simulink model "UNICO"  (R2023b)
settings: Solver=FixedStepDiscrete  StartTime=0.0  StopTime=inf  FixedStep=Control.DT  RelTol=1e-3
values from neighbouring files (symbols this model uses):
  Control =     [Parameters_UNICO.mat]
libraries: simulink x2
(part 3 of 3)

== matlab function UNICO/Wind Speed Estimators/Extended Kalman Filter/GenSpeed_input ==
  data: GenSpMin input; we_inp_speed output; Gearbox_ratio input; RotorSpeed input
function we_inp_speed = fcn(GenSpMin,Gearbox_ratio,RotorSpeed)
% Function to ensure the rotor speed does not fall below a minimum threshold

if RotorSpeed < 0.25*GenSpMin/Gearbox_ratio         % Check if the rotor speed is below 25% of the minimum generator speed, adjusted by the gearbox ratio
    
    we_inp_speed = 0.25*GenSpMin/Gearbox_ratio;     % Set the input speed to the minimum allowable value

else                                                % Otherwise, use the actual rotor speed

    we_inp_speed = RotorSpeed;

end

end

== matlab function UNICO/Pitch Rate Limiter/Rate limiter ==
  data: u_b input; u input; s output; Pitch_Rate input; dt input
function s = fcn(u_b,u,Pitch_Rate, dt)

rate_lim_pos = Pitch_Rate; % rate limit for pitch is simmetric
rate_lim_neg = -Pitch_Rate;

% calculate pitch rate
rate = (u-u_b)/dt;

if rate > rate_lim_pos % if the pitch rate is larger than the maximum allowed, set the pitch using the maximum rate

    s = u_b+rate_lim_pos*dt;

elseif rate < rate_lim_neg % if the pitch rate is smaller than the minimum allowed, set the pitch using the minimum rate

    s = u_b+rate_lim_neg*dt;

else

    s = u;  % if the maximum pitch rate is not violated

end

== matlab function UNICO/Wind Speed Estimators/Extended Kalman Filter/Torque_input ==
  data: GenTorque input; input_torque output; rated_torque input
function input_torque = fcn(GenTorque,rated_torque)
% Function to limit the generator torque to a minimum threshold

if GenTorque < 0.001*rated_torque               % If the generator torque is below 0.001 times the rated torque
    
    input_torque = 0.001*rated_torque;          % Set the input torque to the minimum allowable value

else                                            % Otherwise, use the actual generator torque

    input_torque = GenTorque;

end

end

== matlab function UNICO/Wind Speed Estimators/MATLAB Function ==
  data: WSE_Mode input; TBE_WSpeed input; Raw_WSpeed input; WSpeed output; EKF_WSpeed input
function WSpeed = fcn(WSE_Mode, TBE_WSpeed, Raw_WSpeed, EKF_WSpeed)
if WSE_Mode == 1
    WSpeed = TBE_WSpeed;
elseif WSE_Mode == 2
    WSpeed = EKF_WSpeed;
else
    WSpeed = Raw_WSpeed;
end

== matlab function UNICO/Set Point Smoother/GenSpeed_Ref_Torque_Controller ==
  data: Gen_Ref_torq input; delta_omega input; y output
function y = fcn(Gen_Ref_torq, delta_omega)
% Defining the new generator speed reference for the torque controller

if delta_omega >= 0                     % In Region 2.5 and 3 modify the reference generator speed to avoid conflict with pitch controller

    y = Gen_Ref_torq - delta_omega;     % Following Abbas's rules

else                                    % In Region 2 do no modify the reference generator speed

    y = Gen_Ref_torq;                   

end

end

== matlab function UNICO/Wind Speed Estimators/Extended Kalman Filter/MATLAB Function2 ==
  data: params input; Rot_In output; Radius output; Blade_Height output; Air_Density output; Gearbox_Ratio output; Rated_Torque output; Minimum_Rot_Speed output; Rotor_Area output
function [Rot_In, Radius, Blade_Height, Air_Density, Gearbox_Ratio, Rated_Torque, Minimum_Rot_Speed, Rotor_Area] = fcn(params)
% extracting the generator speed reference   
Radius = params(1); 
Air_Density = params(22);
Blade_Height = params(24);
Rot_In = params(25);
Gearbox_Ratio = params(27);
Rotor_Area = params(28);
Rated_Torque = params(3);
Minimum_Rot_Speed = params(9);
end

== matlab function UNICO/Extract Signals & Filtering/Filtering Block  ==
  data: windNF input; wnd output; wind input; GenSpeedNF input; GenSpeed input; Pitch input; PitchNF input; Tq input; TqNF input; Pwr input; PwrNF input; time input; omega output; ptch output; torque output; Power output; LPF_Starting_Time input
function [wnd,omega,ptch,torque,Power] = fcn(windNF, wind,GenSpeedNF, GenSpeed, Pitch, PitchNF, Tq, TqNF, Pwr, PwrNF, time, LPF_Starting_Time)

% At the beginning of the simulation do not apply filtering to avoid divergence

if time > LPF_Starting_Time

    wnd=wind;        % Wind speed filtered

    omega=GenSpeed;  % Generator speed filtered

    ptch=Pitch;      % Blade picth angle filtered

    torque=Tq;       % Generator torque filtered

    Power=Pwr;       % Generator power filtered

else

    wnd=windNF;         % Wind speed unfiltered

    omega=GenSpeedNF;   % Generator speed unfiltered

    ptch=PitchNF;       % Blade picth angle unfiltered

    torque=TqNF;        % Generator torque unfiltered

    Power=PwrNF;        % Generator power unfiltered

end

== matlab function UNICO/Wind Speed Estimators/Torque Balance Estimator/MATLAB Function2 ==
  data: params input; Rot_In output; Radius output; Blade_Height output; Air_Density output; Gearbox_Ratio output; Rotor_Area output
function [Rot_In, Radius, Blade_Height, Air_Density, Gearbox_Ratio, Rotor_Area]    = fcn(params)
% extracting the generator speed reference 
Radius = params(1); 
Rot_In = params(25);
Blade_Height = params(24);
Air_Density = params(22);
Gearbox_Ratio = params(27);
Rotor_Area = params(28);

end

== matlab function UNICO/Reference Speed Determination/MATLAB Function ==
  data: w0 input; freq input; Ts input; u input; y output
function y = discreteVaryingLowpass(w0, freq, Ts, u)
% DISCRETEVARYINGLOWPASS Implements a 1st-order variable Butterworth filter.
%
% INPUTS:
%   u    : Current input signal
%   freq : Cutoff frequency in rad/s (can vary at each step)
%   Ts   : Sample time in seconds
%   w0   : Pre-warping frequency (rad/s). Set to 0 for standard Tustin.
%
% OUTPUT:
%   y    : Filtered output signal

    % Persistent variables to maintain state between time steps
    persistent u_prev y_prev
    
    % Initialization on the first run
    if isempty(u_prev)
        u_prev = u;
        y_prev = u;
    end

    % --- 1. Pre-warping Gain (K) ---
    % Standard Bilinear (Tustin) transform uses K = 2/Ts.
    % If a pre-warping frequency w0 is provided, K is adjusted.
    if w0 <= 0
        K = 2 / Ts;
    else
        K = w0 / tan(w0 * Ts / 2);
    end

    % --- 2. Variable Coefficient Calculation ---
    % Continuous Transfer Function: H(s) = freq / (s + freq)
    % Substitution: s = K * (z-1) / (z+1)
    
    denominator = (K + freq);
    b0 = freq / denominator;
    b1 = b0;                     % For 1st order Tustin, b0 always equals b1
    a1 = (freq - K) / denominator;

    % --- 3. Difference Equation ---
    % Standard Direct Form I implementation:
    % y[n] = b0*u[n] + b1*u[n-1] - a1*y[n-1]
    y = b0*u + b1*u_prev - a1*y_prev;

    % --- 4. State Update ---
    u_prev = u;
    y_prev = y;
end

== matlab function UNICO/Wind Speed Estimators/Torque Balance Estimator/Torque Balance Estimator LPF ==
  data: w0 input; freq input; Ts input; u input; y output
function y = discreteVaryingLowpass(w0, freq, Ts, u)
% DISCRETEVARYINGLOWPASS Implements a 1st-order variable Butterworth filter.
%
% INPUTS:
%   u    : Current input signal
%   freq : Cutoff frequency in rad/s (can vary at each step)
%   Ts   : Sample time in seconds
%   w0   : Pre-warping frequency (rad/s). Set to 0 for standard Tustin.
%
% OUTPUT:
%   y    : Filtered output signal

    % Persistent variables to maintain state between time steps
    persistent u_prev y_prev
    
    % Initialization on the first run
    if isempty(u_prev)
        u_prev = 0;
        y_prev = 0;
    end

    % --- 1. Pre-warping Gain (K) ---
    % Standard Bilinear (Tustin) transform uses K = 2/Ts.
    % If a pre-warping frequency w0 is provided, K is adjusted.
    if w0 <= 0
        K = 2 / Ts;
    else
        K = w0 / tan(w0 * Ts / 2);
    end

    % --- 2. Variable Coefficient Calculation ---
    % Continuous Transfer Function: H(s) = freq / (s + freq)
    % Substitution: s = K * (z-1) / (z+1)
    
    denominator = (K + freq);
    b0 = freq / denominator;
    b1 = b0;                     % For 1st order Tustin, b0 always equals b1
    a1 = (freq - K) / denominator;

    % --- 3. Difference Equation ---
    % Standard Direct Form I implementation:
    % y[n] = b0*u[n] + b1*u[n-1] - a1*y[n-1]
    y = b0*u + b1*u_prev - a1*y_prev;

    % --- 4. State Update ---
    u_prev = u;
    y_prev = y;
end

== matlab function UNICO/Wind Speed Estimators/Extended Kalman Filter/Extended Kalman Filter LPF ==
  data: w0 input; freq input; Ts input; u input; y output
function y = discreteVaryingLowpass(w0, freq, Ts, u)
% DISCRETEVARYINGLOWPASS Implements a 1st-order variable Butterworth filter.
%
% INPUTS:
%   u    : Current input signal
%   freq : Cutoff frequency in rad/s (can vary at each step)
%   Ts   : Sample time in seconds
%   w0   : Pre-warping frequency (rad/s). Set to 0 for standard Tustin.
%
% OUTPUT:
%   y    : Filtered output signal

    % Persistent variables to maintain state between time steps
    persistent u_prev y_prev
    
    % Initialization on the first run
    if isempty(u_prev)
        u_prev = 0;
        y_prev = 0;
    end

    % --- 1. Pre-warping Gain (K) ---
    % Standard Bilinear (Tustin) transform uses K = 2/Ts.
    % If a pre-warping frequency w0 is provided, K is adjusted.
    if w0 <= 0
        K = 2 / Ts;
    else
        K = w0 / tan(w0 * Ts / 2);
    end

    % --- 2. Variable Coefficient Calculation ---
    % Continuous Transfer Function: H(s) = freq / (s + freq)
    % Substitution: s = K * (z-1) / (z+1)
    
    denominator = (K + freq);
    b0 = freq / denominator;
    b1 = b0;                     % For 1st order Tustin, b0 always equals b1
    a1 = (freq - K) / denominator;

    % --- 3. Difference Equation ---
    % Standard Direct Form I implementation:
    % y[n] = b0*u[n] + b1*u[n-1] - a1*y[n-1]
    y = b0*u + b1*u_prev - a1*y_prev;

    % --- 4. State Update ---
    u_prev = u;
    y_prev = y;
end

== matlab function UNICO/Set Point Smoother/MATLAB Function1 ==
  data: w0 input; freq input; Ts input; u input; y output
function y = discreteVaryingLowpass(w0, freq, Ts, u)
% DISCRETEVARYINGLOWPASS Implements a 1st-order variable Butterworth filter.
%
% INPUTS:
%   u    : Current input signal
%   freq : Cutoff frequency in rad/s (can vary at each step)
%   Ts   : Sample time in seconds
%   w0   : Pre-warping frequency (rad/s). Set to 0 for standard Tustin.
%
% OUTPUT:
%   y    : Filtered output signal

    % Persistent variables to maintain state between time steps
    persistent u_prev y_prev
    
    % Initialization on the first run
    if isempty(u_prev)
        u_prev = 0;
        y_prev = 0;
    end

    % --- 1. Pre-warping Gain (K) ---
    % Standard Bilinear (Tustin) transform uses K = 2/Ts.
    % If a pre-warping frequency w0 is provided, K is adjusted.
    if w0 <= 0
        K = 2 / Ts;
    else
        K = w0 / tan(w0 * Ts / 2);
    end

    % --- 2. Variable Coefficient Calculation ---
    % Continuous Transfer Function: H(s) = freq / (s + freq)
    % Substitution: s = K * (z-1) / (z+1)
    
    denominator = (K + freq);
    b0 = freq / denominator;
    b1 = b0;                     % For 1st order Tustin, b0 always equals b1
    a1 = (freq - K) / denominator;

    % --- 3. Difference Equation ---
    % Standard Direct Form I implementation:
    % y[n] = b0*u[n] + b1*u[n-1] - a1*y[n-1]
    y = b0*u + b1*u_prev - a1*y_prev;

    % --- 4. State Update ---
    u_prev = u;
    y_prev = y;
end

== matlab function UNICO/Set Point Smoother/MATLAB Function2 ==
  data: w0 input; freq input; Ts input; u input; y output
function y = discreteVaryingLowpass(w0, freq, Ts, u)
% DISCRETEVARYINGLOWPASS Implements a 1st-order variable Butterworth filter.
%
% INPUTS:
%   u    : Current input signal
%   freq : Cutoff frequency in rad/s (can vary at each step)
%   Ts   : Sample time in seconds
%   w0   : Pre-warping frequency (rad/s). Set to 0 for standard Tustin.
%
% OUTPUT:
%   y    : Filtered output signal

    % Persistent variables to maintain state between time steps
    persistent u_prev y_prev
    
    % Initialization on the first run
    if isempty(u_prev)
        u_prev = 0;
        y_prev = 0;
    end

    % --- 1. Pre-warping Gain (K) ---
    % Standard Bilinear (Tustin) transform uses K = 2/Ts.
    % If a pre-warping frequency w0 is provided, K is adjusted.
    if w0 <= 0
        K = 2 / Ts;
    else
        K = w0 / tan(w0 * Ts / 2);
    end

    % --- 2. Variable Coefficient Calculation ---
    % Continuous Transfer Function: H(s) = freq / (s + freq)
    % Substitution: s = K * (z-1) / (z+1)
    
    denominator = (K + freq);
    b0 = freq / denominator;
    b1 = b0;                     % For 1st order Tustin, b0 always equals b1
    a1 = (freq - K) / denominator;

    % --- 3. Difference Equation ---
    % Standard Direct Form I implementation:
    % y[n] = b0*u[n] + b1*u[n-1] - a1*y[n-1]
    y = b0*u + b1*u_prev - a1*y_prev;

    % --- 4. State Update ---
    u_prev = u;
    y_prev = y;
end

== matlab function UNICO/Reference Speed Determination/MATLAB Function2 ==
  data: SimTime input; params input; RefSpeedFiltered input; RefSpeedUnfiltered input; Genspeed output
function Genspeed = fcn(SimTime, params, RefSpeedFiltered, RefSpeedUnfiltered)
NF_StartingTime = params(11);

if SimTime > NF_StartingTime
Genspeed = RefSpeedFiltered;
else 
Genspeed =  RefSpeedUnfiltered;
end

== matlab function UNICO/MATLAB Function3 ==
  data: w0 input; freq input; Ts input; u input; y output
function y = discreteVaryingLowpass(w0, freq, Ts, u)
% DISCRETEVARYINGLOWPASS Implements a 1st-order variable Butterworth filter.
%
% INPUTS:
%   u    : Current input signal
%   freq : Cutoff frequency in rad/s (can vary at each step)
%   Ts   : Sample time in seconds
%   w0   : Pre-warping frequency (rad/s). Set to 0 for standard Tustin.
%
% OUTPUT:
%   y    : Filtered output signal

    % Persistent variables to maintain state between time steps
    persistent u_prev y_prev
    
    % Initialization on the first run
    if isempty(u_prev)
        u_prev = 0;
        y_prev = 0;
    end

    % --- 1. Pre-warping Gain (K) ---
    % Standard Bilinear (Tustin) transform uses K = 2/Ts.
    % If a pre-warping frequency w0 is provided, K is adjusted.
    if w0 <= 0
        K = 2 / Ts;
    else
        K = w0 / tan(w0 * Ts / 2);
    end

    % --- 2. Variable Coefficient Calculation ---
    % Continuous Transfer Function: H(s) = freq / (s + freq)
    % Substitution: s = K * (z-1) / (z+1)
    
    denominator = (K + freq);
    b0 = freq / denominator;
    b1 = b0;                     % For 1st order Tustin, b0 always equals b1
    a1 = (freq - K) / denominator;

    % --- 3. Difference Equation ---
    % Standard Direct Form I implementation:
    % y[n] = b0*u[n] + b1*u[n-1] - a1*y[n-1]
    y = b0*u + b1*u_prev - a1*y_prev;

    % --- 4. State Update ---
    u_prev = u;
    y_prev = y;
end

== matlab function UNICO/MATLAB Function4 ==
  data: SimTime input; params input; GenTqFiltered input; GenTqUnfiltered input; GenTq output
function GenTq = fcn(SimTime, params, GenTqFiltered, GenTqUnfiltered)
NF_StartingTime = params(11);

if SimTime > NF_StartingTime
GenTq = GenTqFiltered;
else 
GenTq =  GenTqUnfiltered;
end

== matlab function UNICO/Notch Filter/MATLAB Function2 ==
  data: SimTime input; NFparams input; GenSpeedUnfiltered input; GenSpeedFiltered input; Genspeed output
function Genspeed = fcn(SimTime, NFparams, GenSpeedUnfiltered, GenSpeedFiltered)
NF_StartingTime = NFparams;

if SimTime > NF_StartingTime
Genspeed = GenSpeedFiltered;
else 
Genspeed =  GenSpeedUnfiltered;
end

== matlab function UNICO/Notch Filter/MATLAB Function3 ==
  data: u input; Ts input; f0 input; Filt_GenTq output; zeta_z input; zeta_p input
function Filt_GenTq = notch_filter(u, Ts, f0, zeta_z, zeta_p)

persistent x1 x2 y1 y2 last_f0 last_Ts last_zz last_zp ...
           b0 b1 b2 a1 a2

% Initialize on first run
if isempty(x1)
    x1 = u; x2 = u;
    y1 = u; y2 = u;

    last_f0 = -1;
    last_Ts = -1;
    last_zz = -1;
    last_zp = -1;

    b0 = 1; b1 = 0; b2 = 0;
    a1 = 0; a2 = 0;
end

% Recompute coefficients only when parameters change AND Ts > 0
if (f0 ~= last_f0) || (Ts ~= last_Ts) || ...
   (zeta_z ~= last_zz) || (zeta_p ~= last_zp)

    if Ts > 0
        omega0 = 2*pi*f0;
        K  = 2 / Ts;
        K2 = K * K;
        w2 = omega0 * omega0;

        % Bilinear (Tustin) transform — numerator
        bz0 = K2 + 2*zeta_z*omega0*K + w2;
        bz1 = 2*w2 - 2*K2;
        bz2 = K2 - 2*zeta_z*omega0*K + w2;

        % Bilinear (Tustin) transform — denominator
        az0 = K2 + 2*zeta_p*omega0*K + w2;
        az1 = 2*w2 - 2*K2;
        az2 = K2 - 2*zeta_p*omega0*K + w2;

        % Normalize so a[0] = 1
        b0 = bz0 / az0;
        b1 = bz1 / az0;
        b2 = bz2 / az0;
        a1 = az1 / az0;
        a2 = az2 / az0;
    end
    % Always cache the current parameters (even when Ts=0)
    % so the next call (Ts=dt>0) recomputes correctly
    last_f0 = f0;
    last_Ts = Ts;
    last_zz = zeta_z;
    last_zp = zeta_p;
end

% IIR difference equation
Filt_GenTq = b0*u + b1*x1 + b2*x2 - a1*y1 - a2*y2;

% Update delay states
x2 = x1;
x1 = u;
y2 = y1;
y1 = Filt_GenTq;

end

== matlab function UNICO/Pitch Rate Limiter1/Rate limiter ==
  data: u_b input; u input; s output; Pitch_Rate input; dt input
function s = fcn(u_b, u, Pitch_Rate, dt)
% fcn  Pitch rate limiter (symmetric), all quantities in degrees.
%
%   s = fcn(u_b, u, Pitch_Rate, dt)
%
%   u_b         : previous pitch command [deg]
%   u           : desired (unlimited) pitch command [deg]
%   Pitch_Rate  : maximum allowed pitch rate, given in [rad/s] (symmetric, +/-)
%   dt          : sample time [s]
%   s           : rate-limited pitch command [deg]

rate_lim_pos = Pitch_Rate * (180/pi);     % rate limit for pitch is symmetric [deg/s] (converted from rad/s)
rate_lim_neg = -Pitch_Rate * (180/pi);    % [deg/s]

% calculate pitch rate [deg/s]
rate = (u - u_b) / dt;

if rate > rate_lim_pos
    % if the pitch rate is larger than the maximum allowed, set the pitch using the maximum rate
    s = u_b + rate_lim_pos * dt;
elseif rate < rate_lim_neg
    % if the pitch rate is smaller than the minimum allowed, set the pitch using the minimum rate
    s = u_b + rate_lim_neg * dt;
else
    s = u;  % if the maximum pitch rate is not violated
end

end

== matlab function UNICO/PI CONTROLLER/Gain scheduling ==
  data: GenSpeed input; WindSpeed input; kp_ar input; Ki output; ki_ar input; kp_br input; ki_br input; Kp output; Params input
function [Ki,Kp] = fcn(GenSpeed, WindSpeed, kp_ar, ki_ar,kp_br, ki_br, Params)

R       = Params(1);  % Rotor radius           [m]
v_rt    = Params(2);  % Rated power wind speed [m/s]
w_rt    = Params(5);  % Rated generator speed  [rad/s]
r2      = Params(10);  % Region 2 control mode  {0: optimum tsr tracking; 1: kw^2 torque law}
SpdSwitch = Params(13); %generator speed for switch between region 2 and 2 1/2

% if we use TSR tracking in below rated conditions, schedule the PI
% coefficients
if r2 == 0

    if WindSpeed < v_rt && GenSpeed < w_rt

        % if GenSpeed <=SpdSwitch
        if GenSpeed <= SpdSwitch
            Kp = kp_br;
            Ki = ki_br;

        elseif GenSpeed > SpdSwitch && GenSpeed <w_rt
            % else

            Kp = kp_br+(kp_ar-kp_br)/(w_rt-SpdSwitch)*(GenSpeed-SpdSwitch);
            Ki = ki_br+(ki_ar-ki_br)/(w_rt-SpdSwitch)*(GenSpeed-SpdSwitch);

        else

            Kp = kp_ar;
            Ki = ki_ar;
            % end
        end


    else

        Kp = kp_ar;
        Ki = ki_ar;
    end

else
    % if k-w is used only a set of kp and ki is used
    Kp = kp_ar;
    Ki = ki_ar;

end

== matlab function UNICO/MATLAB Function1 ==
  data: Torque_PI_out input; WindSpeed input; dFPitch input; Pitch_Ctrl_Sw input; Pitch_Controller_Out input; Pitch_out output; params input; Torque_out output
function [Pitch_out, Torque_out] = Pitch_Switch(Torque_PI_out, WindSpeed, dFPitch, Pitch_Ctrl_Sw, Pitch_Controller_Out, params)
v_rt  = params(2);                  % Rated power wind speed [m/s]
dRtTq = params(3);                  % Rated Torque [Nm]

if WindSpeed > v_rt
    if Pitch_Ctrl_Sw == 0
        Pitch_out  = dFPitch * (pi / 180);  % deg → rad
        Torque_out = Torque_PI_out;
    else
        Pitch_out  = Pitch_Controller_Out;
        Torque_out = dRtTq;
    end
else
    Pitch_out  = 0;              % sotto v_rt: passo a zero (fine pitch)
    Torque_out = Torque_PI_out;
end

end

== matlab function UNICO/PI CONTROLLER/Initialize integral term ==
  data: checkDelay input; check output; PI_int input; PI_int output; wg input; WindSpeed input; Architecture_Selector input; Darrieus_Selector input; Params input; propTerm input; T_eq output
function [check,PI_int, T_eq] = fcn(checkDelay, PI_int, wg, WindSpeed, Architecture_Selector, Darrieus_Selector, Params, propTerm)
% Load R struct variables
R       = Params(1);  % Rotor radius                       [m]
v_rt    = Params(2);  % Rated power wind speed             [m/s]
Tq_rated = Params(3); % Rated torque                       [Nm]
w_rt    = Params(5);  % Rated generator speed              [rad/s]
w_min   = Params(9);  % Minimum generator speed            [rad/s]
r2      = Params(10); % Region 2 control mode  {0: optimum tsr tracking; 1: kw^2 torque law}
KSwitch = Params(11); % Region 2 K- switch
Rgn2K = Params(12);   % user defined K value
SpdSwitch = Params(13); %generator speed for switch between region 2 and 2 1/2
w_minSwitch = Params(14); % Switch between region 1.5 and 2 [rad/s]
TSR_opt = Params(15);  % Optimum TSR                             [-]
Cpmax   = Params(16); % max cp value                             [-]
rho     = Params(22);  % Air density                             [kg/m^3]
Bld_Height = Params(24); %Blades Height (VAWT ONLY)              [m]
Rot_area= Params(28); % Rotor Area (VAWT Eggbeater Type ONLY) [m^2]

% Calcola K coerentemente con l'architettura (usato in entrambi i rami r2)
if KSwitch == 1
    K = Rgn2K;
else
    if Architecture_Selector == 1
        K = 0.5*rho*pi*R^5*Cpmax/TSR_opt^3;          % HAWT
    else
        if Darrieus_Selector == 1
            K = rho*R^4*Bld_Height*Cpmax/TSR_opt^3;  % VAWT H-type
        else
            K = 0.5*rho*Rot_area*R^3*Cpmax/TSR_opt^3; % VAWT Eggbeater
        end
    end
end

% ===========================================
% PRIMA: Controlla se siamo in Regione 3
% ===========================================
if WindSpeed > v_rt
    check = 3;
    if checkDelay ~= 3
        % Entrando in Regione 3: inizializza per dare Torque = Torque_rated
        PI_int = Tq_rated - propTerm;
    end

% ===========================================
% ALTRIMENTI: Regione 2 o inferiore
% ===========================================
else
    if r2 == 1
        w1 = SpdSwitch;

        if (wg < w1) && (WindSpeed <= v_rt)
            if wg < w_minSwitch
                % Region 1.5
                check = 15;
                if checkDelay == 2
                    % Venendo da Region 2: inizializza a K*wg^2
                    PI_int = K*wg^2 - propTerm;
                end
                % Se checkDelay == 0: già in 1.5, non toccare
            else
                % Region 2
                check = 2;
            end
        elseif (wg < w_rt) && (WindSpeed <= v_rt)
            % Region 2.5
            check = 25;
            if checkDelay == 2
                % Venendo da Region 2: inizializza a K*wg^2
                PI_int = K*wg^2 - propTerm;
            end
            % checkDelay == 3 o 1: non toccare PI_int
        else
            check = 15;
        end

    else
        % r2 == 0: TSR tracking con PI controller
        check = 2;
        if checkDelay == 0
            % Primo timestep: inizializza PI_int alla coppia di equilibrio
            % usando la stessa formula K*wg^2 del ramo r2==1
            PI_int = K*wg^2 - propTerm;
        end
    end
end

T_eq = K * wg^2;
